simulink model "Narx2Model1"  (R2017a)
settings: Solver=VariableStepAuto  StartTime=0.0  StopTime=500  RelTol=1e-3
settings Model: Creator=Korisnik  LastModifiedBy=Korisnik

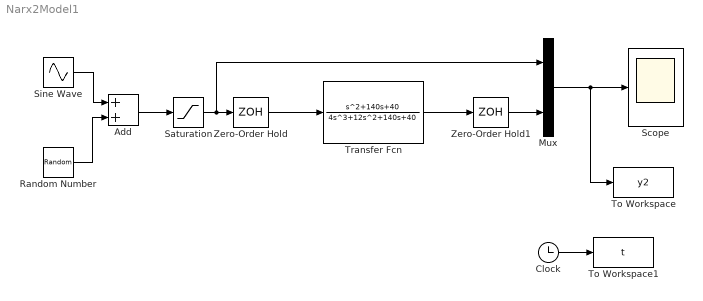
== system Narx2Model1 ==
  Add : Sum
  Clock : Clock
  Mux : Mux  Inputs=2
  Random Number : RandomNumber  Variance=0.1  SampleTime=0.1
  Saturation : Saturate  UpperLimit=5  LowerLimit=-5
  Scope : Scope
  Sine Wave : Sin  Amplitude=4  Frequency=0.025  SampleTime=0.1
  To Workspace : ToWorkspace  VariableName=y2  SampleTime=-1
  To Workspace1 : ToWorkspace  VariableName=t  SaveFormat=Timeseries  SampleTime=-1
  Transfer Fcn : TransferFcn  Numerator=[1 140 40]  Denominator=[4 12 140 40]
  Zero-Order Hold : ZeroOrderHold  SampleTime=0.1
  Zero-Order Hold1 : ZeroOrderHold  SampleTime=0.1
  wires:
  Sine Wave/1 -> Add/1
  Random Number/1 -> Add/2
  Add/1 -> Saturation/1
  Saturation/1 -> Mux/1, Zero-Order Hold/1
  Zero-Order Hold/1 -> Transfer Fcn/1
  Transfer Fcn/1 -> Zero-Order Hold1/1
  Zero-Order Hold1/1 -> Mux/2
  Mux/1 -> To Workspace/1, Scope/1
  Clock/1 -> To Workspace1/1
